simulink model "newmotor"  (R2025a)
settings: Solver=FixedStepDiscrete  StartTime=0.0  StopTime=0.5  FixedStep=Ts  MaxStep=2e-6  EnableMultiTasking=on
PreLoadFcn:
  | assignin('base','Ts',1e-6);
InitFcn:
  | Ts=1e-6;
libraries: spsControlledVoltageSourceLib x2, spsStepperMotorLib x1, spspowerguiLib x1
settings Model: ExtModeAutoUpdateStatusClock=off  Creator=The MathWorks, Inc.  LastModifiedBy=One
settings SolverCC: AlgebraicLoopSolver=TrustRegion
settings DataIOCC: LimitDataPoints=on  SaveFormat=Array  ReturnWorkspaceOutputs=off
settings OptimizationCC: ExpressionDepthLimit=2147483647.0  InitFltsAndDblsToZero=on  LifeSpan=inf
settings DebuggingCC: UnderspecifiedInitializationDetection=Classic  MergeDetectMultiDrivingBlocksExec=none  SignalResolutionControl=TryResolveAllWithWarning  SolverPrmCheckMsg=warning  FcnCallInpInsideContextMsg=warning  UnconnectedInputMsg=warning  UnconnectedOutputMsg=warning  UnconnectedLineMsg=warning  StateNameClashWarn=warning  SubsystemReferenceDiagnosticForUnitTest=warning  SFUnexpectedBacktrackingDiag=warning  SFNoUnconditionalDefaultTransitionDiag=warning  SFExecutionAtInitializationDiag=none  ArithmeticOperatorsInVariantConditions=warning
settings HardwareCC: ProdBitPerPointer=32.0  ProdBitPerSizeT=32.0  ProdBitPerPtrDiffT=32.0  ProdLargestAtomicFloat=None  ProdIntDivRoundTo=Undefined  ProdEndianess=Unspecified  ProdWordSize=32.0  ProdHWDeviceType=32-bit Generic
settings ModelReferenceCC: EnableRefExpFcnMdlSchedulingChecks=on  PropagateSignalLabelsOutOfModel=off
settings SFSimCC: SimUseLocalCustomCode=off  CustomCodeUndefinedFunction=UseInterfaceOnly
settings RTWCC: RTWUseLocalCustomCode=off  GPUComputeCapability=3.5  DLArmComputeVersion=19.05
settings CodeAppCC: StateflowObjectComments=on
settings GRTTargetCC: TargetLangStandard=C89/C90 (ANSI)  CombineOutputUpdateFcns=off  GRTInterface=on
settings ConfigComp: CovMetricSettings=dw  CovSaveCumulativeToWorkspaceVar=on  CovSaveSingleToWorkspaceVar=on  CovExternalEMLEnable=off  CovSFcnEnable=off
settings SimscapeCC: SimscapeNormalizeSystem=off

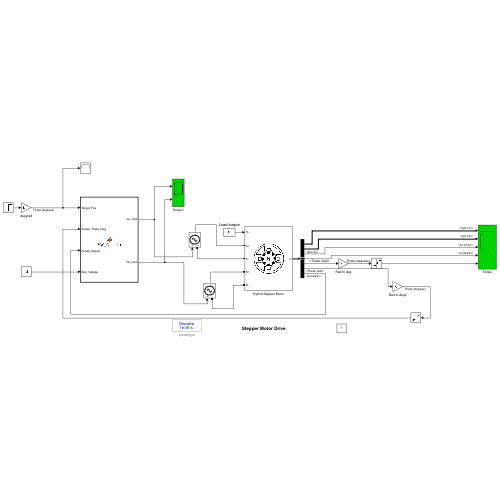
[thumbnail: Simulink's stored preview of the top-level diagram]
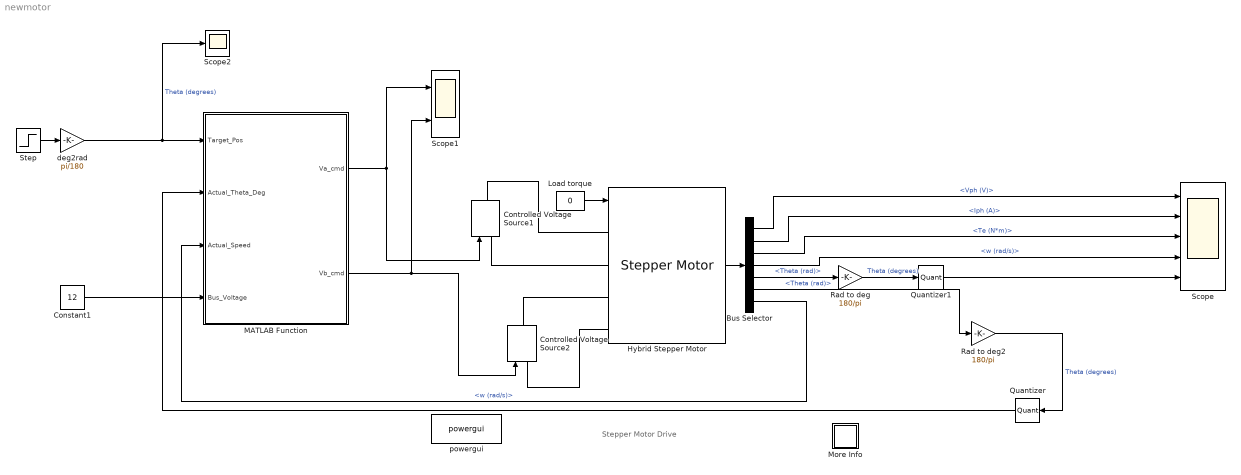
== system newmotor ==
  note: Stepper Motor Drive
  Bus Selector : BusSelector  OutputSignals=Vph (V),Iph (A),Te (N*m),w (rad/s),Theta (rad),Theta (rad),w (rad/s)
  Constant1 : Constant  Value=12
  Controlled Voltage Source1 : spsControlledVoltageSourceLib/Controlled Voltage Source  Initialize=on  Source_Type=AC  Amplitude=0  Phase=0  Frequency=0  Measurements=None
  Controlled Voltage Source2 : spsControlledVoltageSourceLib/Controlled Voltage Source  Initialize=on  Source_Type=AC  Amplitude=0  Phase=0  Frequency=0  Measurements=None
  Hybrid Stepper Motor : spsStepperMotorLib/Stepper Motor  MotorType=Permanent-magnet / Hybrid  NumberOfPhases_1=2  NumberOfPhases_2=3  PresetModel_1=<empty>  PresetModel_2=<empty>  L=1.4e-3  Lmax=10e-3  Lmin=2e-3  R=0.7  Step_angle=1.8  Psim=0.005  Tdm=0.002  J=1.2e-7  B=1e-7*1000  w0=0  pos0=0  TsPowergui=0  TsBlock=-1
  Load torque : Constant  Value=0
  MATLAB Function : MATLAB Function  TreatAsAtomicUnit=on
  More Info : Subsystem
      settings: OpenFcn="showExample(\"simscapeelectricalsps/StepperMotorExample\")"
      mask Display: disp('?')
  Quantizer : Quantizer  QuantizationInterval=360/200/256
  Quantizer1 : Quantizer  QuantizationInterval=360/200/256
  Rad to deg : Gain  Gain=180/pi
  Rad to deg2 : Gain  Gain=180/pi
  Scope : Scope  NumInputPorts=5
      settings: ActiveDisplayYMinimum=-6.23018  ActiveDisplayYMaximum=6.87802  DataLoggingSaveFormat=Array
  Scope1 : Scope  NumInputPorts=2
      settings: ActiveDisplayYMinimum=-30  ActiveDisplayYMaximum=30  DataLoggingSaveFormat=Array
  Scope2 : Scope
      settings: ActiveDisplayYMinimum=2.14159  ActiveDisplayYMaximum=4.14159
  Step : Step  Time=0  After=180  SampleTime=0
  deg2rad : Gain  Gain=pi/180
  powergui : spspowerguiLib/powergui  SimulationMode=Discrete  SampleTime=Ts  frequency=60  Iterations=50  frequencyindice=0  Pbase=100e6  ErrMax=1e-4  UnitsV=kV  UnitsW=MW  buscounter=0  FunctionMessages=off  echomessages=off  EnableUseOfTLC=off  CurrentSourceSwitches=off  DisableSnubberDevices=off  DisableRonSwitches=off  DisableVfSwitches=off  DisplayEquations=off  AutomaticDiscreteSolvers=off  SolverType=Tustin/Backward Euler (TBE)  Interpol=off  ExternalGateDelay=off  methode=off  Ts=0  x0status=blocks  SPID=off  SwTol=0  HookPort=off  NonlinearTolerance=1e-4  nMaxIteration=100  ContinueOnMaxIteration=off  RestoreLinks=warning  ResistiveCurrentMeasurement=off  Frange=[0:2:500]  Ylog=off  Xlog=on  ShowGrid=off  save=off  variable=ZData  structure=0  ZoomFFT=on  StartTime=0.0  cycles=1  DisplayStyle=1  fundamental=60  FreqAxis=off  MaxFrequency=1000  frequencyindicesteady=1  RmsSteady=1  display=off
  wires:
  Load torque/1 -> Hybrid Stepper Motor/1
  Hybrid Stepper Motor/1 -> Bus Selector/1
  Bus Selector/1 -> Scope/1  "<Vph (V)>"
  Bus Selector/2 -> Scope/2  "<Iph (A)>"
  Bus Selector/3 -> Scope/3  "<Te (N*m)>"
  Bus Selector/4 -> Scope/4  "<w (rad/s)>"
  Rad to deg/1 -> Quantizer1/1  "Theta (degrees)"
  Bus Selector/5 -> Rad to deg/1  "<Theta (rad)>"
  Bus Selector/6 -> Rad to deg2/1  "<Theta (rad)>"
  MATLAB Function/1(Va_cmd) -> Scope1/1, Controlled Voltage Source1/1
  MATLAB Function/2(Vb_cmd) -> Controlled Voltage Source2/1, Scope1/2
  deg2rad/1 -> Scope2/1, MATLAB Function/1(Target_Pos)  "Theta (degrees)"
  Constant1/1 -> MATLAB Function/4(Bus_Voltage)
  Bus Selector/7 -> MATLAB Function/3(Actual_Speed)  "<w (rad/s)>"
  Step/1 -> deg2rad/1
  Rad to deg2/1 -> Quantizer/1  "Theta (degrees)"
  Quantizer/1 -> MATLAB Function/2(Actual_Theta_Deg)
  Quantizer1/1 -> Scope/5
  connections:
  Controlled Voltage Source1/RConn1 -- Hybrid Stepper Motor/LConn1
  Controlled Voltage Source1/LConn1 -- Hybrid Stepper Motor/LConn2
  Controlled Voltage Source2/RConn1 -- Hybrid Stepper Motor/LConn3
  Controlled Voltage Source2/LConn1 -- Hybrid Stepper Motor/LConn4

== system newmotor/More Info ==

== matlab function newmotor/MATLAB Function ==
  data: Target_Pos input; Va_cmd output; Actual_Theta_Deg input; Actual_Speed input; Bus_Voltage input; Vb_cmd output
function [Va_cmd, Vb_cmd] = FOC_Controller(Target_Pos, Actual_Theta_Deg, Actual_Speed, Bus_Voltage)
    % =========================================================================
    %  FOC 闭环控制器 (含 PID + 前馈补偿)
    % =========================================================================
    
    % --- 1. 参数设置 (根据仿真表现微调) ---
    PolePairs   = 50;     % 极对数 (1.8度步进电机 = 50)
    Max_Current = 2.0;    % 最大允许电流 (A)
    
    % [核心参数调优]
    % 增大 Kp 提高响应速度，增大 Kv 消除震荡
    Kp_pos = 100.0;        % 位置环 P (刚度)
    Kv_pos = 0.3;         % 速度环 D (阻尼)
    
    % [前馈参数]
    % 反电动势常数 Ke (Volts / (rad/s))
    % 经验值：如果不确定，可以设为 0.05 到 0.1 之间试一试
    Ke = 0.08;            
    
    % 模拟电流环增益 (假设 V = I * R_equivalent)
    % 因为没有模拟真实的电流环PI，这里用一个比例系数代替
    Current_Gain = 1.5;   

    % --- 2. 数据预处理 ---
    % 将机械角度 (度) 转换为 机械弧度
    Theta_mech_rad = Actual_Theta_Deg * (pi/180);
    
    % 将机械弧度 转换为 电角度 (用于 FOC 变换)
    Theta_elec = Theta_mech_rad * PolePairs;
    
    % --- 3. 控制律计算 (PID 部分) ---
    % 计算位置误差
    Pos_Error = Target_Pos - Theta_mech_rad;
    
    % PD 控制器计算目标力矩电流 (Iq)
    % 逻辑：I_target = (误差 * P) - (速度 * D)
    I_target = Pos_Error * Kp_pos - Actual_Speed * Kv_pos;
    
    % 电流限幅 (保护电机)
    if I_target > Max_Current
        I_target = Max_Current;
    elseif I_target < -Max_Current
        I_target = -Max_Current;
    end

% --- 4. 坐标变换 (FOC 核心 - 加 90 度写法) ---
    % 目标：生成与转子磁场正交(Q轴)的电流矢量
    
    % [物理含义对应]
    % C++ 代码: focPosition = estPosition + 256; 
    % Simulink: Theta_foc = Theta_elec + (pi / 2);
    % 这里的 (pi/2) 就对应了固件里的 256 步
    
    Theta_foc = Theta_elec + (pi / 2); 
    
    % 直接投影到 Alpha-Beta 坐标系
    % Alpha = I * cos(Angle)
    % Beta  = I * sin(Angle)
    
    I_alpha = I_target * cos(Theta_foc);
    I_beta  = I_target * sin(Theta_foc);
    

    % --- 5. 前馈补偿 (Feed-Forward) ---
    % 计算反电动势 (Back-EMF)
    % 电机转得越快，反电动势越大，会抵消驱动电压
    % 我们在这里提前把这部分电压加上去
    
    % V_bemf_q = Speed * Ke (Q轴方向的反电动势)
    % 将其变换到 Alpha-Beta 坐标系
    V_bemf_alpha = -Actual_Speed * Ke * sin(Theta_elec);
    V_bemf_beta  =  Actual_Speed * Ke * cos(Theta_elec);
    
    % --- 6. 最终输出计算 ---
    % 输出电压 = (PID计算电流 * 增益) + 前馈补偿
    Va_raw = (I_alpha * Current_Gain) + V_bemf_alpha;
    Vb_raw = (I_beta  * Current_Gain) + V_bemf_beta;
    
    % --- 7. 电压限幅 (SVPWM 范围限制) ---
    % 限制输出电压不超过母线电压
    if Va_raw > Bus_Voltage, Va_cmd = Bus_Voltage; 
    elseif Va_raw < -Bus_Voltage, Va_cmd = -Bus_Voltage;
    else, Va_cmd = Va_raw;
    end
    
    if Vb_raw > Bus_Voltage, Vb_cmd = Bus_Voltage;
    elseif Vb_raw < -Bus_Voltage, Vb_cmd = -Bus_Voltage;
    else, Vb_cmd = Vb_raw;
    end
    
end
